simulink model "exp2_bilateral_nodelay_stg2"  (R2025a)
settings: Solver=ode4  StartTime=0.0  StopTime=10.0  RelTol=1e-3
values from neighbouring files (symbols this model uses):
  Ts = T(T.classCode == 0,:)    [exp2_sweep_final.m]
undefined symbols (not defined in the file or in its folder): a, b_eq, Bc, I_eq, k_eq, Kc, r_h, r_m, r_s, vM0, vS0, xM0, xS0
settings Model: Creator=ekaitz  LastModifiedBy=ekaitz

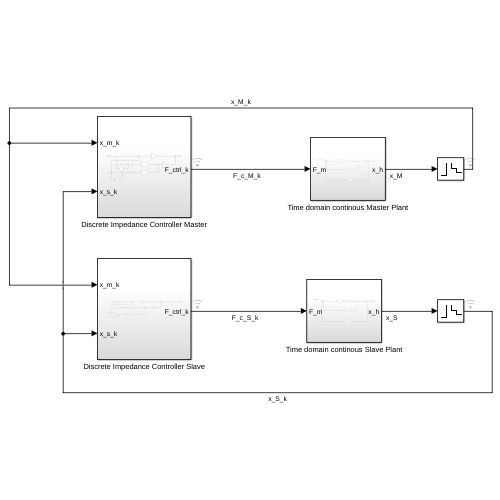
[thumbnail: Simulink's stored preview of the top-level diagram]
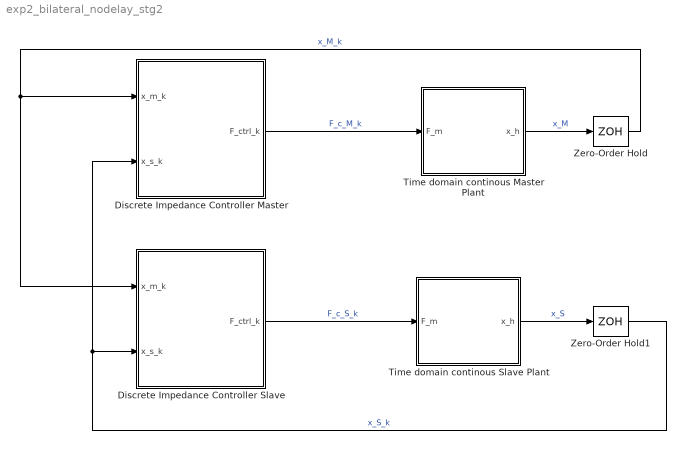
== system exp2_bilateral_nodelay_stg2 ==
  Discrete Impedance Controller Master : Subsystem
  Discrete Impedance Controller Slave : Subsystem
  Time domain continous Master Plant : Subsystem
  Time domain continous Slave Plant : Subsystem
  Zero-Order Hold : ZeroOrderHold  SampleTime=Ts
  Zero-Order Hold1 : ZeroOrderHold  SampleTime=Ts
  wires:
  Time domain continous Slave Plant/1(x_h) -> Zero-Order Hold1/1  "x_S"
  Time domain continous Master Plant/1(x_h) -> Zero-Order Hold/1  "x_M"
  Discrete Impedance Controller Master/1(F_ctrl_k) -> Time domain continous Master Plant/1(F_m)  "F_c_M_k"
  Discrete Impedance Controller Slave/1(F_ctrl_k) -> Time domain continous Slave Plant/1(F_m)  "F_c_S_k"
  Zero-Order Hold1/1 -> Discrete Impedance Controller Slave/2(x_s_k), Discrete Impedance Controller Master/2(x_s_k)  "x_S_k"
  Zero-Order Hold/1 -> Discrete Impedance Controller Slave/1(x_m_k), Discrete Impedance Controller Master/1(x_m_k)  "x_M_k"

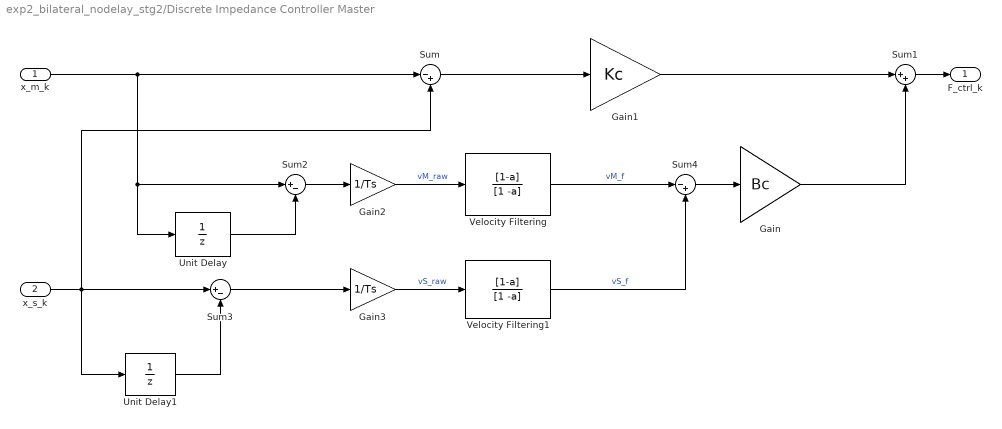
== system exp2_bilateral_nodelay_stg2/Discrete Impedance Controller Master ==
  x_m_k : Inport
  x_s_k : Inport  Port=2
  Gain : Gain  Gain=Bc
  Gain1 : Gain  Gain=Kc
  Gain2 : Gain  Gain=1/Ts
  Gain3 : Gain  Gain=1/Ts
  Sum : Sum  Inputs=|-+
  Sum1 : Sum  Inputs=|++
  Sum2 : Sum  Inputs=|+-
  Sum3 : Sum  Inputs=|+-
  Sum4 : Sum  Inputs=|-+
  Unit Delay : UnitDelay  InitialCondition=xM0  SampleTime=Ts  HasFrameUpgradeWarning=on
  Unit Delay1 : UnitDelay  InitialCondition=xS0  SampleTime=Ts  HasFrameUpgradeWarning=on
  Velocity Filtering : DiscreteTransferFcn  Numerator=[1-a]  Denominator=[1 -a]
  Velocity Filtering1 : DiscreteTransferFcn  Numerator=[1-a]  Denominator=[1 -a]
  F_ctrl_k : Outport
  wires:
  Sum/1 -> Gain1/1
  Gain1/1 -> Sum1/1
  Gain/1 -> Sum1/2
  Sum1/1 -> F_ctrl_k/1
  x_m_k/1 -> Sum2/1, Unit Delay/1, Sum/1
  Unit Delay/1 -> Sum2/2
  Sum2/1 -> Gain2/1
  Sum3/1 -> Gain3/1
  Unit Delay1/1 -> Sum3/2
  x_s_k/1 -> Sum3/1, Sum/2, Unit Delay1/1
  Gain2/1 -> Velocity Filtering/1  "vM_raw"
  Gain3/1 -> Velocity Filtering1/1  "vS_raw"
  Velocity Filtering/1 -> Sum4/1  "vM_f"
  Velocity Filtering1/1 -> Sum4/2  "vS_f"
  Sum4/1 -> Gain/1

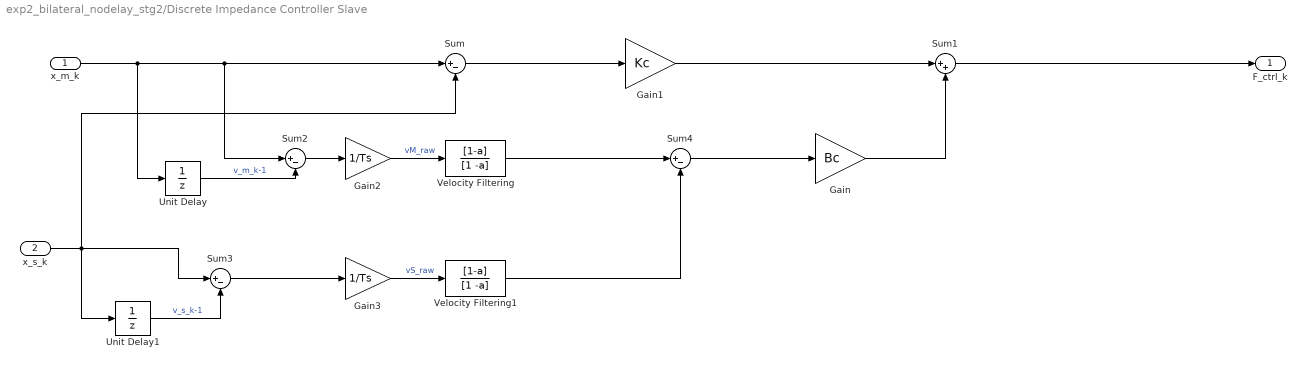
== system exp2_bilateral_nodelay_stg2/Discrete Impedance Controller Slave ==
  x_m_k : Inport
  x_s_k : Inport  Port=2
  Gain : Gain  Gain=Bc
  Gain1 : Gain  Gain=Kc
  Gain2 : Gain  Gain=1/Ts
  Gain3 : Gain  Gain=1/Ts
  Sum{,2..4} (4 alike) : Sum  Inputs=|+-
  Sum1 : Sum  Inputs=|++
  Unit Delay : UnitDelay  InitialCondition=xM0  SampleTime=Ts  HasFrameUpgradeWarning=on
  Unit Delay1 : UnitDelay  InitialCondition=xS0  SampleTime=Ts  HasFrameUpgradeWarning=on
  Velocity Filtering : DiscreteTransferFcn  Numerator=[1-a]  Denominator=[1 -a]
  Velocity Filtering1 : DiscreteTransferFcn  Numerator=[1-a]  Denominator=[1 -a]
  F_ctrl_k : Outport
  wires:
  Sum/1 -> Gain1/1
  Gain1/1 -> Sum1/1
  Gain/1 -> Sum1/2
  Sum1/1 -> F_ctrl_k/1
  x_m_k/1 -> Unit Delay/1, Sum2/1, Sum/1
  Unit Delay/1 -> Sum2/2  "v_m_k-1"
  Sum2/1 -> Gain2/1
  Sum3/1 -> Gain3/1
  Unit Delay1/1 -> Sum3/2  "v_s_k-1"
  x_s_k/1 -> Sum3/1, Sum/2, Unit Delay1/1
  Gain2/1 -> Velocity Filtering/1  "vM_raw"
  Gain3/1 -> Velocity Filtering1/1  "vS_raw"
  Velocity Filtering/1 -> Sum4/1
  Velocity Filtering1/1 -> Sum4/2
  Sum4/1 -> Gain/1

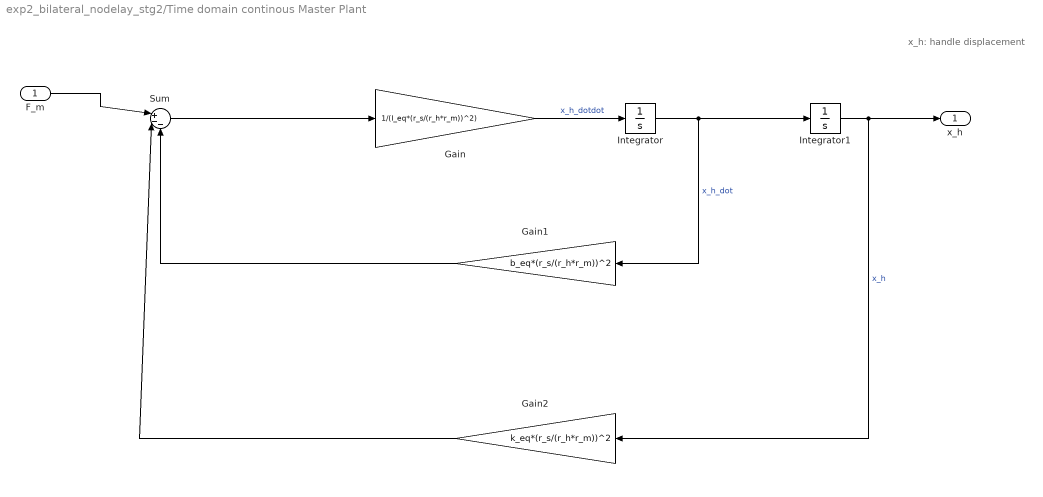
== system exp2_bilateral_nodelay_stg2/Time domain continous Master Plant ==
  note: x_h: handle displacement
  F_m : Inport
  Gain : Gain  Gain=1/(I_eq*(r_s/(r_h*r_m))^2)
  Gain1 : Gain  Gain=b_eq*(r_s/(r_h*r_m))^2
  Gain2 : Gain  Gain=k_eq*(r_s/(r_h*r_m))^2
  Integrator : Integrator  InitialCondition=vM0
  Integrator1 : Integrator  InitialCondition=xM0
  Sum : Sum  Inputs=|+--
  x_h : Outport
  wires:
  Gain2/1 -> Sum/2
  Gain/1 -> Integrator/1  "x_h_dotdot"
  F_m/1 -> Sum/1
  Integrator1/1 -> x_h/1, Gain2/1  "x_h"
  Gain1/1 -> Sum/3
  Sum/1 -> Gain/1
  Integrator/1 -> Gain1/1, Integrator1/1  "x_h_dot"

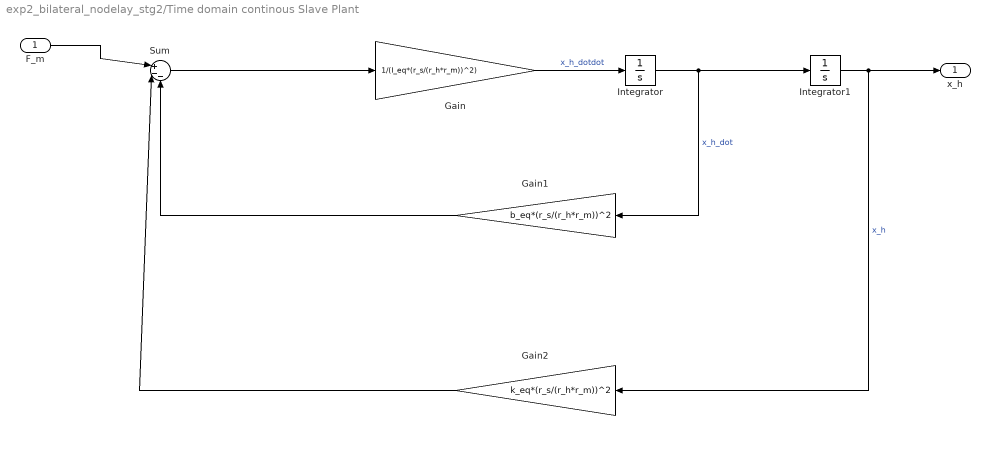
== system exp2_bilateral_nodelay_stg2/Time domain continous Slave Plant ==
  F_m : Inport
  Gain : Gain  Gain=1/(I_eq*(r_s/(r_h*r_m))^2)
  Gain1 : Gain  Gain=b_eq*(r_s/(r_h*r_m))^2
  Gain2 : Gain  Gain=k_eq*(r_s/(r_h*r_m))^2
  Integrator : Integrator  InitialCondition=vS0
  Integrator1 : Integrator  InitialCondition=xS0
  Sum : Sum  Inputs=|+--
  x_h : Outport
  wires:
  Gain2/1 -> Sum/2
  Gain/1 -> Integrator/1  "x_h_dotdot"
  F_m/1 -> Sum/1
  Integrator1/1 -> x_h/1, Gain2/1  "x_h"
  Gain1/1 -> Sum/3
  Sum/1 -> Gain/1
  Integrator/1 -> Gain1/1, Integrator1/1  "x_h_dot"
